simulink model "Crusier_system_os"  (R2023b)
settings: Solver=FixedStepDiscrete  StartTime=0.0  StopTime=inf  FixedStep=1  RelTol=1e-3
(part 2 of 2)

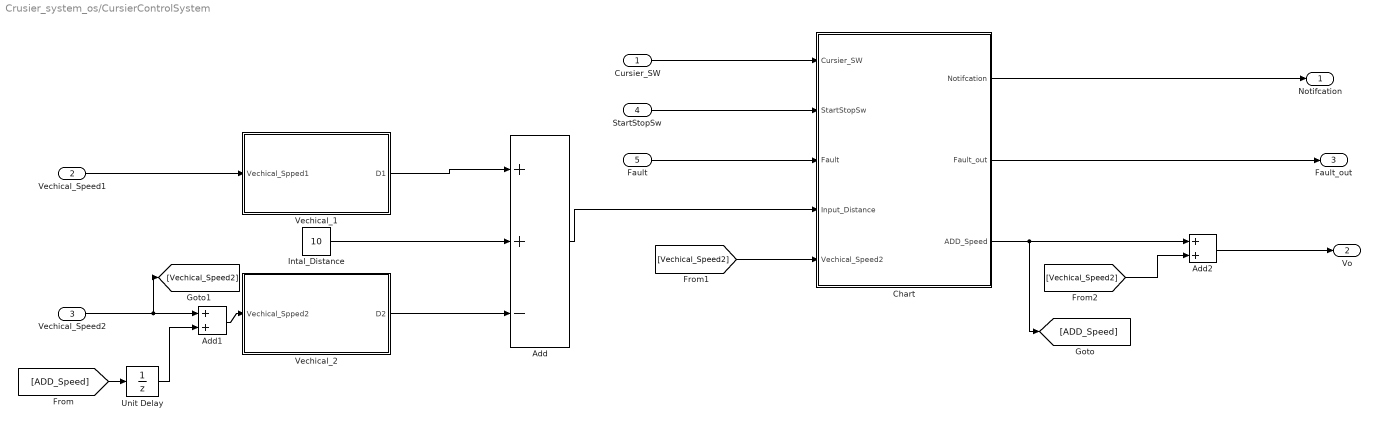
== system Crusier_system_os/CursierControlSystem ==
  Cursier_SW : Inport
  Vechical_Speed1 : Inport  Port=2
  Vechical_Speed2 : Inport  Port=3
  StartStopSw : Inport  Port=4
  Fault : Inport  Port=5
  Add : Sum  Inputs=++-
  Add1 : Sum
  Add2 : Sum
  Chart : Stateflow chart  TreatAsAtomicUnit=on
  Intal_Distance : Constant  Value=10
  Unit Delay : UnitDelay  SampleTime=-1  HasFrameUpgradeWarning=on
  Vechical_1 : Subsystem
      mask Display: image('Vechical1.png')
  Vechical_2 : Subsystem
      mask Display: image('Vechical2.png')
  Notifcation : Outport
  Vo : Outport  Port=2
  Fault_out : Outport  Port=3
  wires:
  Cursier_SW/1 -> Chart/1(Cursier_SW)
  StartStopSw/1 -> Chart/2(StartStopSw)
  Fault/1 -> Chart/3(Fault)
  Chart/3(ADD_Speed) -> [ADD_Speed], Add2/1
  Chart/1(Notifcation) -> Notifcation/1
  Chart/2(Fault_out) -> Fault_out/1
  Add/1 -> Chart/4(Input_Distance)
  Vechical_Speed2/1 -> [Vechical_Speed2], Add1/1
  Vechical_Speed1/1 -> Vechical_1/1(Vechical_Spped1)
  Intal_Distance/1 -> Add/2
  Vechical_1/1(D1) -> Add/1
  Vechical_2/1(D2) -> Add/3
  Add1/1 -> Vechical_2/1(Vechical_Spped2)
  [ADD_Speed] -> Unit Delay/1
  [Vechical_Speed2] -> Chart/5(Vechical_Speed2)
  Add2/1 -> Vo/1
  [Vechical_Speed2] -> Add2/2
  Unit Delay/1 -> Add1/2

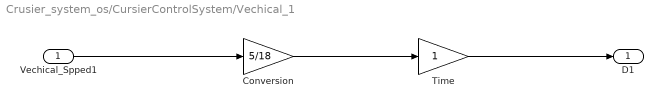
== system Crusier_system_os/CursierControlSystem/Vechical_1 ==
  Vechical_Spped1 : Inport
  Conversion : Gain  Gain=5/18
  Time : Gain
  D1 : Outport
  wires:
  Vechical_Spped1/1 -> Conversion/1
  Conversion/1 -> Time/1
  Time/1 -> D1/1

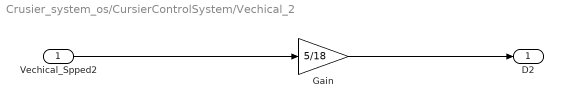
== system Crusier_system_os/CursierControlSystem/Vechical_2 ==
  Vechical_Spped2 : Inport
  Gain : Gain  Gain=5/18
  D2 : Outport
  wires:
  Gain/1 -> D2/1
  Vechical_Spped2/1 -> Gain/1

== stateflow chart Crusier_system_os/CursierControlSystem/Chart ==
  state Regular_System [parallel]
    settings: executionOrder=1
    state Cruiser_On
      state Modes
        state Fault_Send
          en:
          Notifcation=Car_Modes.Fault;
          send(Fault_event,FaultDetection);
        state Accelerate
          en:
          Notifcation=Car_Modes.Accelerate;
          ADD_Speed=ADD_Speed+5;
          du:
          ADD_Speed=ADD_Speed+5;
        state Decelerate
          en:
          Notifcation=Car_Modes.Decelerate;
          ADD_Speed=ADD_Speed-5;
          du:
          ADD_Speed=ADD_Speed-10;
        state Do_Nothing
          en:
          Notifcation=Car_Modes.Do_Nothing;
        state Stop
          en:
          Notifcation=Car_Modes.Stop;
          ADD_Speed=-Vechical_Speed2;
          du:
          ADD_Speed=-Vechical_Speed2;
        state brake
          en:
          Notifcation=Car_Modes.brake;
          ADD_Speed=-Vechical_Speed2+5;
          du:
          ADD_Speed=-Vechical_Speed2+5;
        (default) -> Accelerate
        (junction 29) -> Fault_Send [order 2] : [Fault==1]
        Fault_Send -> (junction 29) : [Fault==0]
        Accelerate -> (junction 29)
        (junction 29) -> Accelerate [order 4] : [Input_Distance>15]
        Decelerate -> (junction 29)
        (junction 29) -> Decelerate [order 5] : [Input_Distance<10]
        brake -> (junction 29)
        (junction 29) -> brake [order 3] : [Input_Distance<5]
        Stop -> (junction 29)
        (junction 29) -> Stop [order 1] : [Input_Distance<1.5]
        Do_Nothing -> (junction 29)
        (junction 29) -> Do_Nothing [order 6] : [(5<Input_Distance)&&(Input_Distance<10)]
      (default) -> Modes
    state Cruiser_Off
      en:
      Notifcation=Car_Modes.Cruiser_Off;
    (default) -> Cruiser_On
    Cruiser_On -> Cruiser_Off : [(Cursier_SW==OFF)||(StartStopSw==ON)]
    Cruiser_Off -> Cruiser_On [order 2] : [(Cursier_SW==ON)&&(StartStopSw==OFF)]
    (junction 62) -> Cruiser_Off : {send(Fault_event,FaultDetection)}
    Cruiser_Off -> (junction 62) [order 1] : [Fault==1]
  state FaultDetection [parallel]
    settings: executionOrder=2
    state Non_Fault
      en:
      Fault_out=0;
    state Fault
      en:
      Fault_out=1;
    state meduim
    (default) -> Non_Fault
    Non_Fault -> meduim : Fault_event{Notifcation=Car_Modes.Fault}
    meduim -> Fault : after(5,sec)
  data: Notifcation output; Fault_out output double; Cursier_SW input; StartStopSw input; Fault input; ADD_Speed output =0; OFF local double =0; ON local double =1; Input_Distance input double; Vechical_Speed2 input
  events: Fault_event local FUNCTION_CALL_EVENT
